simulink model "White_Activity8"  (R2020b)
settings: Solver=VariableStepAuto  StartTime=0.0  StopTime=10.0  RelTol=1e-3
settings Model: Creator=Michael  LastModifiedBy=Michael
settings OptimizationCC: BlockReduction=off  DefaultParameterBehavior=Inlined  BufferReuse=off

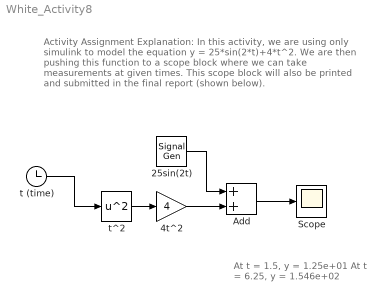
== system White_Activity8 ==
  note: At t = 1.5, y = 1.25e+01
      | At t = 6.25, y = 1.546e+02
  note: Activity Assignment Explanation:
      | In this activity, we are using only simulink to model the equation y = 25*sin(2*t)+4*t^2. We are then pushing this function to a scope block where we can take measurements at given times. This scope block will also be printed and submitted in the final report (shown below).
  25sin(2t) : SignalGenerator  Amplitude=25  Frequency=2  Units=rad/sec
  4t^2 : Gain  Gain=4
  Add : Sum
  Scope : Scope
  t (time) : Clock
  t^2 : Math  Operator=square  SignedPower=on  RndMeth=Zero  SaturateOnIntegerOverflow=on
  wires:
  t (time)/1 -> t^2/1
  t^2/1 -> 4t^2/1
  4t^2/1 -> Add/2
  25sin(2t)/1 -> Add/1
  Add/1 -> Scope/1
